simulink model "task3"  (R2025b)
settings: Solver=VariableStepAuto  StartTime=0.0  StopTime=24  RelTol=1e-3
values from neighbouring files (symbols this model uses):
  Pf = 1.5    [init.m]
  Pr = 7.0    (= 7)    [init.m]
  Sb_0 = 0.55    [init.m]
  Ta_0 = 10.0    (= 10)    [init.m]
  Tp_0 = 11.5    [init.m]
  Ts = 0.1    [init.m]    (also in run_task7.m = Ts_vec(k))
libraries: slpidlib x2
settings Model: Creator=davide  LastModifiedBy=davide

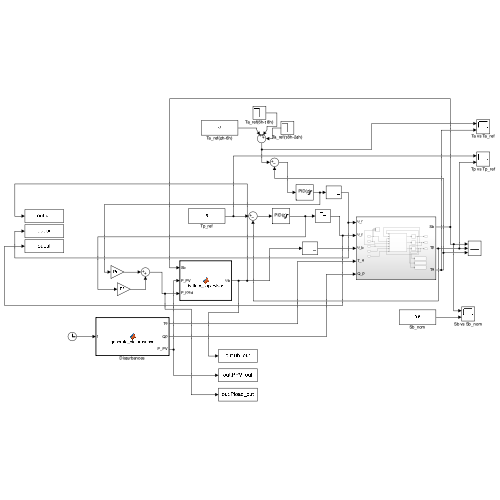
[thumbnail: Simulink's stored preview of the top-level diagram]
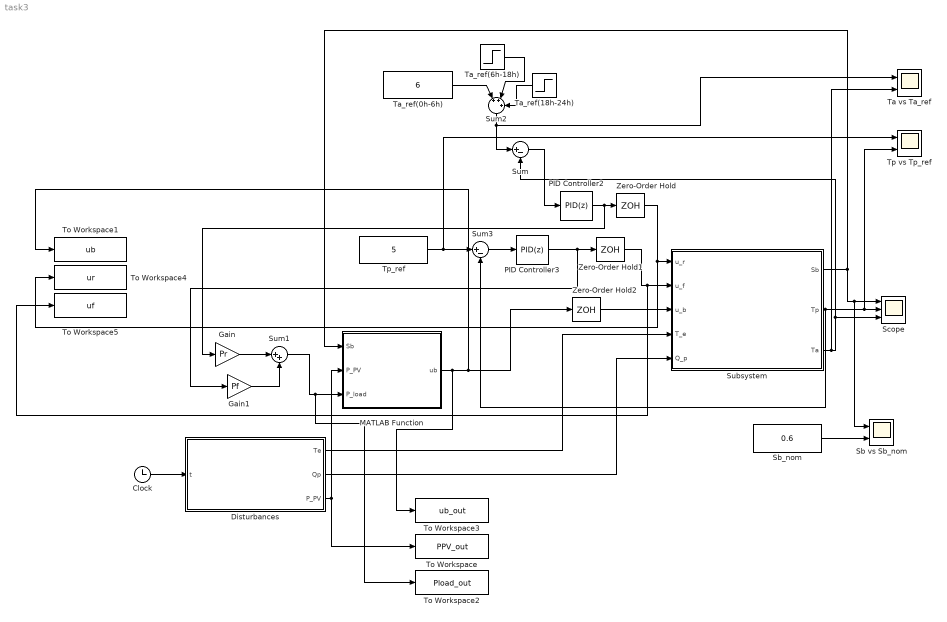
== system task3 ==
  Clock : Clock
  Disturbances : MATLAB Function  TreatAsAtomicUnit=on
  Gain : Gain  Gain=Pr
  Gain1 : Gain  Gain=Pf
  MATLAB Function : MATLAB Function  TreatAsAtomicUnit=on
  PID Controller2 : slpidlib/PID Controller  Controller=PID  Form=Parallel  TimeDomain=Discrete-time  UseExternalTs=off  SampleTime=Ts  IntegratorMethod=Forward Euler  FilterMethod=Forward Euler  ControllerParametersSource=internal  P=-0.05  I=-0.025  UseKiTs=off  D=0  UseExternalDerivativeSource=off  N=100  UseFilter=on  TunerSelectOption=Transfer Function Based (PID Tuner App)  InitialConditionSource=internal  InitialConditionForIntegrator=0  InitialConditionForFilter=0  DifferentiatorICPrevScaledInput=0  ExternalReset=none  TrackingMode=off  Kt=1  LimitOutput=on  SatLimitsSource=internal  UpperSaturationLimit=1  LowerSaturationLimit=0  LinearizeAsGain=on  AntiWindupMode=back-calculation  Kb=1  LimitIntegrator=off  UpperIntegratorSaturationLimit=inf  LowerIntegratorSaturationLimit=-inf  POutMin=[]  POutMax=[]  IOutMin=[]  IOutMax=[]  DOutMin=[]  DOutMax=[]  NOutMin=[]  NOutMax=[]  SumOutMin=[]  SumOutMax=[]  SaturationOutMin=[]  SaturationOutMax=[]  PParamMin=[]  PParamMax=[]  IParamMin=[]  IParamMax=[]  DParamMin=[]  DParamMax=[]  NParamMin=[]  NParamMax=[]  KbParamMin=[]  KbParamMax=[]  KtParamMin=[]  KtParamMax=[]  KbOutMin=[]  KbOutMax=[]  KtOutMin=[]  KtOutMax=[]  IntegratorOutMin=[]  IntegratorOutMax=[]  FilterOutMin=[]  FilterOutMax=[]  SumI1OutMin=[]  SumI1OutMax=[]  SumI2OutMin=[]  SumI2OutMax=[]  SumI3OutMin=[]  SumI3OutMax=[]  SumI4OutMin=[]  SumI4OutMax=[]  SumDOutMin=[]  SumDOutMax=[]  DifferentiatorOutMin=[]  DifferentiatorOutMax=[]  FilterDiffOutCoefMin=[]  FilterDiffOutCoefMax=[]  ReciprocalOutMin=[]  ReciprocalOutMax=[]  SumDenOutMin=[]  SumDenOutMax=[]  SumNumOutMin=[]  SumNumOutMax=[]  DivideOutMin=[]  DivideOutMax=[]  UdiffTsProdOutMin=[]  UdiffTsProdOutMax=[]  NTsProdOutMin=[]  NTsProdOutMax=[]  UintegralTsProdOutMin=[]  UintegralTsProdOutMax=[]  UngainTsProdOutMin=[]  UngainTsProdOutMax=[]  ClampingZeroOutDataTypeStr=Inherit: Inherit via back propagation  ClampingZeroOutMin=[]  ClampingZeroOutMax=[]  FilterDenConstantOutDataTypeStr=Inherit: Inherit via back propagation  FilterDenConstantOutMin=[]  FilterDenConstantOutMax=[]  PCopyOutDataTypeStr=Inherit: Inherit via back propagation  PCopyOutMin=[]  PCopyOutMax=[]  NCopyOutDataTypeStr=Inherit: Inherit via back propagation  NCopyOutMin=[]  NCopyOutMax=[]  IntegratorContinuousStateAttributes=''  IntegratorStateMustResolveToSignalObject=off  IntegratorRTWStateStorageClass=Auto  FilterContinuousStateAttributes=''  FilterStateMustResolveToSignalObject=off  FilterRTWStateStorageClass=Auto  ParallelPVariant=InternalParameters  IdealPVariant=Disabled  IVariant=InternalParameters  DVariant=InternalParameters  IntegratorVariant=Discrete  SatVariant=Enabled  AWVariant=BackCalculation  PCopyVariant=Disabled  TRVariant=Disabled  FdbkBlocksVariant=Forward  IdealPFdbkVariant=Disabled  SatFdbkVariant=Disabled  DerivativeFilterVariant=ForwardEulerFilter  NVariant=InternalParameters  NCopyVariant=Disabled  FilterICVariant=InternalICsFilter  IntegratorICVariant=InternalICs  ExternalResetVariant=Disabled  TRSumVariant=Passthrough  SumFdbkVariant=Disabled  SumVariant=Sum_PID  TsampFilterVariant=InternalTs  TsampNgainVariant=Passthrough  TsampIntegralVariant=Disabled_SignalSpec  ExternalSaturationOutDataTypeStr=Inherit: Same as second input  DerivativeSourceVariant=ErrorSignal  PreIntVariant=InternalPreInt
  PID Controller3 : slpidlib/PID Controller  Controller=PID  Form=Parallel  TimeDomain=Discrete-time  UseExternalTs=off  SampleTime=Ts  IntegratorMethod=Forward Euler  FilterMethod=Forward Euler  ControllerParametersSource=internal  P=-0.05  I=-0.025  UseKiTs=off  D=0  UseExternalDerivativeSource=off  N=100  UseFilter=on  TunerSelectOption=Transfer Function Based (PID Tuner App)  InitialConditionSource=internal  InitialConditionForIntegrator=0  InitialConditionForFilter=0  DifferentiatorICPrevScaledInput=0  ExternalReset=none  TrackingMode=off  Kt=1  LimitOutput=on  SatLimitsSource=internal  UpperSaturationLimit=1  LowerSaturationLimit=0  LinearizeAsGain=on  AntiWindupMode=back-calculation  Kb=1  LimitIntegrator=off  UpperIntegratorSaturationLimit=inf  LowerIntegratorSaturationLimit=-inf  POutMin=[]  POutMax=[]  IOutMin=[]  IOutMax=[]  DOutMin=[]  DOutMax=[]  NOutMin=[]  NOutMax=[]  SumOutMin=[]  SumOutMax=[]  SaturationOutMin=[]  SaturationOutMax=[]  PParamMin=[]  PParamMax=[]  IParamMin=[]  IParamMax=[]  DParamMin=[]  DParamMax=[]  NParamMin=[]  NParamMax=[]  KbParamMin=[]  KbParamMax=[]  KtParamMin=[]  KtParamMax=[]  KbOutMin=[]  KbOutMax=[]  KtOutMin=[]  KtOutMax=[]  IntegratorOutMin=[]  IntegratorOutMax=[]  FilterOutMin=[]  FilterOutMax=[]  SumI1OutMin=[]  SumI1OutMax=[]  SumI2OutMin=[]  SumI2OutMax=[]  SumI3OutMin=[]  SumI3OutMax=[]  SumI4OutMin=[]  SumI4OutMax=[]  SumDOutMin=[]  SumDOutMax=[]  DifferentiatorOutMin=[]  DifferentiatorOutMax=[]  FilterDiffOutCoefMin=[]  FilterDiffOutCoefMax=[]  ReciprocalOutMin=[]  ReciprocalOutMax=[]  SumDenOutMin=[]  SumDenOutMax=[]  SumNumOutMin=[]  SumNumOutMax=[]  DivideOutMin=[]  DivideOutMax=[]  UdiffTsProdOutMin=[]  UdiffTsProdOutMax=[]  NTsProdOutMin=[]  NTsProdOutMax=[]  UintegralTsProdOutMin=[]  UintegralTsProdOutMax=[]  UngainTsProdOutMin=[]  UngainTsProdOutMax=[]  ClampingZeroOutDataTypeStr=Inherit: Inherit via back propagation  ClampingZeroOutMin=[]  ClampingZeroOutMax=[]  FilterDenConstantOutDataTypeStr=Inherit: Inherit via back propagation  FilterDenConstantOutMin=[]  FilterDenConstantOutMax=[]  PCopyOutDataTypeStr=Inherit: Inherit via back propagation  PCopyOutMin=[]  PCopyOutMax=[]  NCopyOutDataTypeStr=Inherit: Inherit via back propagation  NCopyOutMin=[]  NCopyOutMax=[]  IntegratorContinuousStateAttributes=''  IntegratorStateMustResolveToSignalObject=off  IntegratorRTWStateStorageClass=Auto  FilterContinuousStateAttributes=''  FilterStateMustResolveToSignalObject=off  FilterRTWStateStorageClass=Auto  ParallelPVariant=InternalParameters  IdealPVariant=Disabled  IVariant=InternalParameters  DVariant=InternalParameters  IntegratorVariant=Discrete  SatVariant=Enabled  AWVariant=BackCalculation  PCopyVariant=Disabled  TRVariant=Disabled  FdbkBlocksVariant=Forward  IdealPFdbkVariant=Disabled  SatFdbkVariant=Disabled  DerivativeFilterVariant=ForwardEulerFilter  NVariant=InternalParameters  NCopyVariant=Disabled  FilterICVariant=InternalICsFilter  IntegratorICVariant=InternalICs  ExternalResetVariant=Disabled  TRSumVariant=Passthrough  SumFdbkVariant=Disabled  SumVariant=Sum_PID  TsampFilterVariant=InternalTs  TsampNgainVariant=Passthrough  TsampIntegralVariant=Disabled_SignalSpec  ExternalSaturationOutDataTypeStr=Inherit: Same as second input  DerivativeSourceVariant=ErrorSignal  PreIntVariant=InternalPreInt
  Sb vs Sb_nom : Scope  NumInputPorts=2
      settings: ActiveDisplayYMinimum=0.53745740515106444  ActiveDisplayYMaximum=0.66288335364042017  DataLoggingVariableName=ScopeData4
  Sb_nom : Constant  Value=0.6
  Scope : Scope  NumInputPorts=3
      settings: ActiveDisplayYMinimum=-1.2186402756478434  ActiveDisplayYMaximum=12.91318225284976
  Subsystem : Subsystem
  Sum : Sum  Inputs=|+-
  Sum1 : Sum  Inputs=|++
  Sum2 : Sum  Inputs=|+++
  Sum3 : Sum  Inputs=|+-
  Ta vs Ta_ref : Scope  NumInputPorts=2
      settings: ActiveDisplayYMinimum=1.8570700267652394  ActiveDisplayYMaximum=11.639529708174706  DataLoggingVariableName=ScopeData2
  Ta_ref(0h-6h) : Constant  Value=6
  Ta_ref(18h-24h) : Step  Time=18  After=-1  SampleTime=0
  Ta_ref(6h-18h) : Step  Time=6  After=-1  SampleTime=0
  To Workspace : ToWorkspace  VariableName=PPV_out  SampleTime=-1
      settings: Save2DSignal=2-D array (concatenate along first dimension)
  To Workspace1 : ToWorkspace  VariableName=ub  SaveFormat=Timeseries  SampleTime=-1
      settings: Save2DSignal=2-D array (concatenate along first dimension)
  To Workspace2 : ToWorkspace  VariableName=Pload_out  SampleTime=-1
      settings: Save2DSignal=2-D array (concatenate along first dimension)
  To Workspace3 : ToWorkspace  VariableName=ub_out  SampleTime=-1
      settings: Save2DSignal=2-D array (concatenate along first dimension)
  To Workspace4 : ToWorkspace  VariableName=ur  SaveFormat=Timeseries  SampleTime=-1
      settings: Save2DSignal=2-D array (concatenate along first dimension)
  To Workspace5 : ToWorkspace  VariableName=uf  SaveFormat=Timeseries  SampleTime=-1
      settings: Save2DSignal=2-D array (concatenate along first dimension)
  Tp vs Tp_ref : Scope  NumInputPorts=2
      settings: ActiveDisplayYMinimum=1.8570700267652394  ActiveDisplayYMaximum=11.639529708174706  DataLoggingVariableName=ScopeData3
  Tp_ref : Constant  Value=5
  Zero-Order Hold : ZeroOrderHold  SampleTime=Ts
  Zero-Order Hold1 : ZeroOrderHold  SampleTime=Ts
  Zero-Order Hold2 : ZeroOrderHold  SampleTime=Ts
  wires:
  Clock/1 -> Disturbances/1(t)
  Disturbances/1(Te) -> Subsystem/4(T_e)
  Disturbances/2(Qp) -> Subsystem/5(Q_p)
  Subsystem/3(Ta) -> Ta vs Ta_ref/2, Sum/2, Scope/3
  Subsystem/2(Tp) -> Tp vs Tp_ref/2, Scope/2, Sum3/2
  Subsystem/1(Sb) -> Sb vs Sb_nom/1, Scope/1, MATLAB Function/1(Sb)
  Ta_ref(18h-24h)/1 -> Sum2/3
  Ta_ref(6h-18h)/1 -> Sum2/2
  Ta_ref(0h-6h)/1 -> Sum2/1
  Sum2/1 -> Ta vs Ta_ref/1, Sum/1
  Sum/1 -> PID Controller2/1
  PID Controller2/1 -> Gain/1, Zero-Order Hold/1
  Tp_ref/1 -> Tp vs Tp_ref/1, Sum3/1
  Sum3/1 -> PID Controller3/1
  MATLAB Function/1(ub) -> To Workspace3/1, To Workspace1/1, Zero-Order Hold2/1
  Disturbances/3(P_PV) -> MATLAB Function/2(P_PV), To Workspace/1
  Gain1/1 -> Sum1/2
  Gain/1 -> Sum1/1
  Sum1/1 -> To Workspace2/1, MATLAB Function/3(P_load)
  Zero-Order Hold/1 -> To Workspace4/1, Subsystem/1(u_r)
  Zero-Order Hold1/1 -> To Workspace5/1, Subsystem/2(u_f)
  PID Controller3/1 -> Gain1/1, Zero-Order Hold1/1
  Zero-Order Hold2/1 -> Subsystem/3(u_b)
  Sb_nom/1 -> Sb vs Sb_nom/2

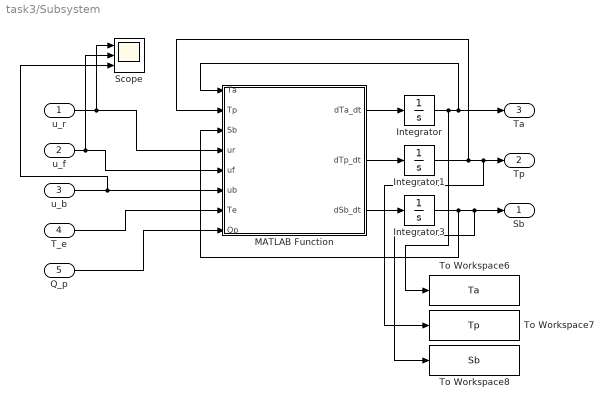
== system task3/Subsystem ==
  u_r : Inport
  u_f : Inport  Port=2
  u_b : Inport  Port=3
  T_e : Inport  Port=4
  Q_p : Inport  Port=5
  Integrator : Integrator  InitialCondition=Ta_0
  Integrator1 : Integrator  InitialCondition=Tp_0
  Integrator3 : Integrator  InitialCondition=Sb_0
  MATLAB Function : MATLAB Function  TreatAsAtomicUnit=on
  Scope : Scope  NumInputPorts=3
  To Workspace6 : ToWorkspace  VariableName=Ta  SaveFormat=Timeseries  SampleTime=-1
      settings: Save2DSignal=2-D array (concatenate along first dimension)
  To Workspace7 : ToWorkspace  VariableName=Tp  SaveFormat=Timeseries  SampleTime=-1
      settings: Save2DSignal=2-D array (concatenate along first dimension)
  To Workspace8 : ToWorkspace  VariableName=Sb  SaveFormat=Timeseries  SampleTime=-1
      settings: Save2DSignal=2-D array (concatenate along first dimension)
  Sb : Outport
  Tp : Outport  Port=2
  Ta : Outport  Port=3
  wires:
  MATLAB Function/1(dTa_dt) -> Integrator/1
  MATLAB Function/2(dTp_dt) -> Integrator1/1
  MATLAB Function/3(dSb_dt) -> Integrator3/1
  Integrator3/1 -> To Workspace8/1, Sb/1, MATLAB Function/3(Sb)
  Integrator/1 -> To Workspace6/1, Ta/1, MATLAB Function/1(Ta)
  Integrator1/1 -> MATLAB Function/2(Tp), To Workspace7/1, Tp/1
  u_r/1 -> Scope/1, MATLAB Function/4(ur)
  u_b/1 -> Scope/3, MATLAB Function/6(ub)
  T_e/1 -> MATLAB Function/7(Te)
  Q_p/1 -> MATLAB Function/8(Qp)
  u_f/1 -> MATLAB Function/5(uf), Scope/2

== matlab function task3/Disturbances ==
  data: t input; Te output; Qp output; P_PV output
function [Te, Qp, P_PV] = generate_disturbances(t)
    Rmax = 850; Pmax = 9.0;
    
    Te = 24 + 8 * sin(pi/12 * (t - 8));
    
    if t >= 6 && t <= 18
        Rs = Rmax * sin(pi * (t - 6) / 12);
    else
        Rs = 0;
    end
    P_PV = Pmax * (Rs / Rmax);
    
    % Thermal Charge   
    if t < 4
        Qp = 1200;
    elseif t < 10
        Qp = 600;
    else
        Qp = 250;
    end
end

== matlab function task3/Subsystem/MATLAB Function ==
  data: Ta input; dTa_dt output; Tp input; Sb input; ur input; uf input; ub input; Te input; Qp input; dTp_dt output; dSb_dt output
function [dTa_dt, dTp_dt, dSb_dt] = plant_equations(Ta, Tp, Sb, ur, uf, ub, Te, Qp)
    Ca = 1.5e5; Cp = 8.0e5; ke = 3.8*70; kr = 1.6e4; kf = 450; alpha_f = 1.0;
    Eb = 18; eta_b = 0.94; sec2hour = 3600;

    % Saturations
    ur = max(0, min(1, ur));
    uf = max(0, min(1, uf));
    ub = max(-4, min(4, ub));
    
    if (Sb <= 0.15 && ub < 0) || (Sb >= 0.95 && ub > 0)
        ub = 0; 
    end

    % sec2hour
    dTa_dt = (sec2hour / Ca) * (ke * (Te - Ta) - kr * ur - kf * (1 + alpha_f * uf) * (Ta - Tp) + Qp);
    dTp_dt = (sec2hour / Cp) * (kf * (1 + alpha_f * uf) * (Ta - Tp));
    dSb_dt = (1 / Eb) * ( eta_b * max(-ub, 0) - (1 / eta_b) * max(ub, 0) );
end

== matlab function task3/MATLAB Function ==
  data: Sb input; ub output; P_PV input; P_load input
function ub = battery_supervisor(Sb, P_PV, P_load)
    Sb_nom = 0.60;
    ub_max =  4.0;
    ub_min = -4.0;
    Kb = 100;  % compromesso: abbastanza grande da correggere SOC,
              % abbastanza piccolo da non bloccare la scarica notturna
    
    P_net = P_load - P_PV;

    % Feedforward: copri il deficit/surplus
    ub_ff = P_net;

    % Correzione SOC proporzionale
    P_soc = Kb * (Sb - Sb_nom);

    ub_req = ub_ff + P_soc;

    % Carica SOLO con surplus PV
    if ub_req < 0 && P_net >= 0
        ub_req = 0;
    end

    % Non caricare oltre il surplus disponibile
    if ub_req < 0 && P_net < 0
        ub_req = max(ub_req, P_net);
    end

    % Limiti SOC
    if Sb <= 0.20 && ub_req > 0
        ub_req = 0;
    elseif Sb >= 0.90 && ub_req < 0
        ub_req = 0;
    end

    ub = max(ub_min, min(ub_max, ub_req));
end
